simulink model "Robot_DH_FK"  (R2023b)
settings: Solver=VariableStepAuto  StartTime=0.0  StopTime=10.0  RelTol=1e-3
values from neighbouring files (symbols this model uses):
  a1 = 40    [FK.m]    (also in IK_Analytical.m = 0.04; IK_MDH.m = 0.04; IK_Position.m = 0.04; IK_Solver.m = 0.04)
  a2 = 275    [FK.m]    (also in IK_Analytical.m = 0.275; IK_MDH.m = 0.275; IK_Position.m = 0.275; IK_Solver.m = 0.275)
  a3 = 25    [FK.m]    (also in IK_Analytical.m = 0.025; IK_MDH.m = 0.025; IK_Position.m = 0.025; IK_Solver.m = 0.025)
  d1 = 342    [FK.m]    (also in IK_Analytical.m = 0.342; IK_MDH.m = 0.342; IK_Position.m = 0.342; IK_Solver.m = 0.342)
  d4 = 280    [FK.m]    (also in IK_Analytical.m = 0.28; IK_MDH.m = 0.28; IK_Position.m = 0.28; IK_Solver.m = 0.28)
  fc1 = 0    [set_mode_parameter.m]
  fc2 = 0    [set_mode_parameter.m]
  fc3 = 0    [set_mode_parameter.m]
  fc4 = 0    [set_mode_parameter.m]
  fc5 = 0    [set_mode_parameter.m]
  fc6 = 0    [set_mode_parameter.m]
  fv1 = 0    [set_mode_parameter.m]
  fv2 = 0    [set_mode_parameter.m]
  fv3 = 0    [set_mode_parameter.m]
  fv4 = 0    [set_mode_parameter.m]
  fv5 = 0    [set_mode_parameter.m]
  fv6 = 0    [set_mode_parameter.m]
  Ia1 = 0    [set_mode_parameter.m]
  Ia2 = 0    [set_mode_parameter.m]
  Ia3 = 0    [set_mode_parameter.m]
  Ia4 = 0    [set_mode_parameter.m]
  Ia5 = 0    [set_mode_parameter.m]
  Ia6 = 0    [set_mode_parameter.m]
  Ic111 = 0    [set_mode_parameter.m]
  Ic112 = 0    [set_mode_parameter.m]
  Ic113 = 0    [set_mode_parameter.m]
  Ic122 = 0    [set_mode_parameter.m]
  Ic123 = 0    [set_mode_parameter.m]
  Ic133 = 1.3676    [set_mode_parameter.m]
  Ic211 = 8.8194    [set_mode_parameter.m]
  Ic212 = 0    [set_mode_parameter.m]
  Ic213 = 0    [set_mode_parameter.m]
  Ic222 = 6.0549    [set_mode_parameter.m]
  Ic223 = 0    [set_mode_parameter.m]
  Ic233 = 0.9569    [set_mode_parameter.m]
  Ic311 = 0.0332    [set_mode_parameter.m]
  Ic312 = 0    [set_mode_parameter.m]
  Ic313 = 0    [set_mode_parameter.m]
  Ic322 = 1.8442    [set_mode_parameter.m]
  Ic323 = 0    [set_mode_parameter.m]
  Ic333 = 1.0560    (= 1.056)    [set_mode_parameter.m]
  Ic411 = 0.1448    [set_mode_parameter.m]
  Ic412 = 0    [set_mode_parameter.m]
  Ic413 = 0    [set_mode_parameter.m]
  Ic422 = 0.0015    [set_mode_parameter.m]
  Ic423 = 0    [set_mode_parameter.m]
  Ic433 = 0.0822    [set_mode_parameter.m]
  Ic511 = 0    [set_mode_parameter.m]
  Ic512 = 0    [set_mode_parameter.m]
  Ic513 = 0    [set_mode_parameter.m]
  Ic522 = 0.0121    [set_mode_parameter.m]
  Ic523 = 0    [set_mode_parameter.m]
  Ic533 = 0.0299    [set_mode_parameter.m]
  Ic611 = 0.0134    [set_mode_parameter.m]
  Ic612 = 0    [set_mode_parameter.m]
  Ic613 = 0    [set_mode_parameter.m]
  Ic622 = 0    [set_mode_parameter.m]
  Ic623 = 0    [set_mode_parameter.m]
  Ic633 = 0.0051    [set_mode_parameter.m]
  m = (c1*px + s1*py) - dt*(c1*ax + s1*ay) - a1    [IK_6DOF_Robot.m]    (also in IK_MDH.m = pwx_1 - a1; IK_MDH_Robot.m = rho - a1)
  m1 = 0.167    [set_mode_parameter.m]
  m2 = 1    [set_mode_parameter.m]
  m3 = 0.5    [set_mode_parameter.m]
  m4 = 0.333    [set_mode_parameter.m]
  m5 = 0.25    [set_mode_parameter.m]
  m6 = 0.2    [set_mode_parameter.m]
  mc11 = 0    [set_mode_parameter.m]
  mc12 = 0    [set_mode_parameter.m]
  mc13 = 0.2    [set_mode_parameter.m]
  mc21 = 0.1291    [set_mode_parameter.m]
  mc22 = 0    [set_mode_parameter.m]
  mc23 = 3.3117    [set_mode_parameter.m]
  mc31 = 1.6484    [set_mode_parameter.m]
  mc32 = 0    [set_mode_parameter.m]
  mc33 = 0.8748    [set_mode_parameter.m]
  mc41 = 0.3200    (= 0.32)    [set_mode_parameter.m]
  mc42 = 0.2324    [set_mode_parameter.m]
  mc43 = 0.7083    [set_mode_parameter.m]
  mc51 = 0.4574    [set_mode_parameter.m]
  mc52 = 0    [set_mode_parameter.m]
  mc53 = 0.6427    [set_mode_parameter.m]
  mc61 = 0.3200    (= 0.32)    [set_mode_parameter.m]
  mc62 = -0.0513    [set_mode_parameter.m]
  mc63 = 0.6417    [set_mode_parameter.m]
  MDH = [ ... (first row only)    [FK_MDH.m]    (also in optimize_MDH_params.m = [x(1:6), [0; 0; 0.275; 0.025; 0; 0],         [0.342; 0.040; ; set_mode_parameter.m; test_222.m)
  N = size(waypoints, 2)    [run_trajectory.m]
  s = zc - d(1)    [inverse_kinematics_6dof.m]
  XB4 = SerialLink([L1 L2 L3 L4 L5 L6], 'name', 'XB4')    [Toolbox_Motheds_1.m]
undefined symbols (not defined in the file or in its folder): X, Y, Z
libraries: sm_lib x56, nesl_utility x31, simulink_extras x2, simulink x2, robotcorelib x1
(part 2 of 2)

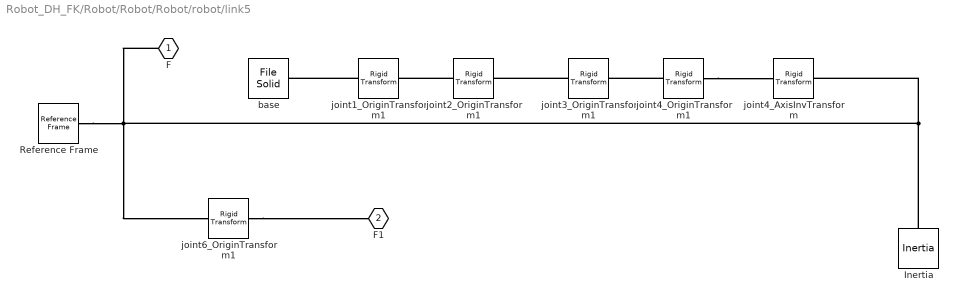
== system Robot_DH_FK/Robot/Robot/Robot/robot/link5 ==
  Inertia : sm_lib/Body Elements/Inertia  InertiaType=Custom  Mass=m5  MassUnits=kg  CenterOfMass=[mc51 mc52 mc53]  CenterOfMassUnits=m  MomentsOfInertia=[Ic511 Ic522 Ic533]  MomentsOfInertiaUnits=kg*m^2  ProductsOfInertia=[Ic523 Ic513 Ic512]  ProductsOfInertiaUnits=kg*m^2  GraphicType=Marker  MarkerShape=Inertia  MarkerSize=20  GraphicVisPropType=SimpleVisualProperties  GraphicDiffuseColor=[0.5 0.5 0.5]  GraphicSpecularColor=[0.5 0.5 0.5 1.0]  GraphicAmbientColor=[0.15 0.15 0.15 1.0]  GraphicEmissiveColor=[0.0 0.0 0.0 1.0]  GraphicShininess=75  GraphicOpacity=1.0
  Reference Frame : sm_lib/Frames and Transforms/Reference Frame
  base : sm_lib/Body Elements/File Solid  ExtGeomFileName=/home/jiehuang/Documents/Custom-Robot/Matlab_Study/Matlab2023Project/IntroductionBook/程序/XB4模型/XB4-5.STL  UnitType=Custom  ExtGeomFileUnits=mm  StepReaderType=HEX  ExportConvexHullGeometry=off  InertiaType=Custom  Mass=0  MassUnits=kg  CenterOfMass=[0 0 0]  CenterOfMassUnits=m  MomentsOfInertia=[0 0 0]  MomentsOfInertiaUnits=kg*m^2  ProductsOfInertia=[0 0 0]  ProductsOfInertiaUnits=kg*m^2  BasedOnType=Density  Density=1000  DensityUnits=kg/(m^3)  DoExposeReferenceFrame=on  SerializedFrames=<Frames/>  GraphicType=FromGeometry  MarkerShape=Sphere  MarkerSize=10  GraphicVisPropType=SimpleVisualProperties  GraphicDiffuseColor=[0.5 0.5 0.5]  GraphicSpecularColor=[0.5 0.5 0.5 1.0]  GraphicAmbientColor=[0.15 0.15 0.15 1.0]  GraphicEmissiveColor=[0.0 0.0 0.0 1.0]  GraphicShininess=75  GraphicOpacity=1.0
  joint1_OriginTransform1 : sm_lib/Frames and Transforms/Rigid Transform  TranslationMethod=Cartesian  TranslationStandardOffset=0  TranslationStandardOffsetUnits=m  TranslationStandardAxis=+Z  TranslationCartesianOffset=[0 0 d1]  TranslationCartesianOffsetUnits=m  TranslationROffset=0  TranslationROffsetUnits=m  TranslationZOffset=0  TranslationZOffsetUnits=m  TranslationThetaOffset=0  TranslationThetaOffsetUnits=deg  RotationMethod=RotationSequence  RotationAngleUnits=deg  RotationStandardAxis=+Z  RotationAngle=0.0  RotationArbitraryAxis=[0 0 1]  FollAlignAxisA=+X  BaseAlignAxisA=+Y  FollAlignAxisB=+Y  BaseAlignAxisB=+Z  RotationSequenceAxes=BaseAxes  RotationSequence=XYZ  RotationSequenceAngles=[0 0 0]  RotationSequenceAnglesUnits=rad  RotationMatrix=[1 0 0; 0 1 0; 0 0 1]  Quaternion=[1 0 0 0]
  joint2_OriginTransform1 : sm_lib/Frames and Transforms/Rigid Transform  TranslationMethod=Cartesian  TranslationStandardOffset=0  TranslationStandardOffsetUnits=m  TranslationStandardAxis=+Z  TranslationCartesianOffset=[a1 0 0]  TranslationCartesianOffsetUnits=m  TranslationROffset=0  TranslationROffsetUnits=m  TranslationZOffset=0  TranslationZOffsetUnits=m  TranslationThetaOffset=0  TranslationThetaOffsetUnits=deg  RotationMethod=RotationSequence  RotationAngleUnits=deg  RotationStandardAxis=+Z  RotationAngle=0.0  RotationArbitraryAxis=[0 0 1]  FollAlignAxisA=+X  BaseAlignAxisA=+Y  FollAlignAxisB=+Y  BaseAlignAxisB=+Z  RotationSequenceAxes=FollowerAxes  RotationSequence=XYZ  RotationSequenceAngles=[-pi/2 0 -pi/2]  RotationSequenceAnglesUnits=rad  RotationMatrix=[1 0 0; 0 1 0; 0 0 1]  Quaternion=[1 0 0 0]
  joint3_OriginTransform1 : sm_lib/Frames and Transforms/Rigid Transform  TranslationMethod=Cartesian  TranslationStandardOffset=0  TranslationStandardOffsetUnits=m  TranslationStandardAxis=+Z  TranslationCartesianOffset=[a2 0 0]  TranslationCartesianOffsetUnits=m  TranslationROffset=0  TranslationROffsetUnits=m  TranslationZOffset=0  TranslationZOffsetUnits=m  TranslationThetaOffset=0  TranslationThetaOffsetUnits=deg  RotationMethod=RotationSequence  RotationAngleUnits=deg  RotationStandardAxis=+Z  RotationAngle=0.0  RotationArbitraryAxis=[0 0 1]  FollAlignAxisA=+X  BaseAlignAxisA=+Y  FollAlignAxisB=+Y  BaseAlignAxisB=+Z  RotationSequenceAxes=FollowerAxes  RotationSequence=XYZ  RotationSequenceAngles=[0 0 0]  RotationSequenceAnglesUnits=rad  RotationMatrix=[1 0 0; 0 1 0; 0 0 1]  Quaternion=[1 0 0 0]
  joint4_AxisInvTransform : sm_lib/Frames and Transforms/Rigid Transform  TranslationMethod=Cartesian  TranslationStandardOffset=0  TranslationStandardOffsetUnits=m  TranslationStandardAxis=+Z  TranslationCartesianOffset=[0 0 0]  TranslationCartesianOffsetUnits=m  TranslationROffset=0  TranslationROffsetUnits=m  TranslationZOffset=0  TranslationZOffsetUnits=m  TranslationThetaOffset=0  TranslationThetaOffsetUnits=deg  RotationMethod=RotationSequence  RotationAngleUnits=rad  RotationStandardAxis=+Z  RotationAngle=1.570796  RotationArbitraryAxis=[0 1 0]  FollAlignAxisA=+X  BaseAlignAxisA=+Y  FollAlignAxisB=+Y  BaseAlignAxisB=+Z  RotationSequenceAxes=FollowerAxes  RotationSequence=XYZ  RotationSequenceAngles=[pi/2 0 0]  RotationSequenceAnglesUnits=rad  RotationMatrix=[1 0 0; 0 1 0; 0 0 1]  Quaternion=[1 0 0 0]
  joint4_OriginTransform1 : sm_lib/Frames and Transforms/Rigid Transform  TranslationMethod=Cartesian  TranslationStandardOffset=0  TranslationStandardOffsetUnits=m  TranslationStandardAxis=+Z  TranslationCartesianOffset=[a3 d4 0]  TranslationCartesianOffsetUnits=m  TranslationROffset=0  TranslationROffsetUnits=m  TranslationZOffset=0  TranslationZOffsetUnits=m  TranslationThetaOffset=0  TranslationThetaOffsetUnits=deg  RotationMethod=RotationSequence  RotationAngleUnits=deg  RotationStandardAxis=+Z  RotationAngle=0.0  RotationArbitraryAxis=[0 0 1]  FollAlignAxisA=+X  BaseAlignAxisA=+Y  FollAlignAxisB=+Y  BaseAlignAxisB=+Z  RotationSequenceAxes=FollowerAxes  RotationSequence=XYZ  RotationSequenceAngles=[-pi/2 0 0]  RotationSequenceAnglesUnits=rad  RotationMatrix=[1 0 0; 0 1 0; 0 0 1]  Quaternion=[1 0 0 0]
  joint6_OriginTransform1 : sm_lib/Frames and Transforms/Rigid Transform  TranslationMethod=Cartesian  TranslationStandardOffset=0  TranslationStandardOffsetUnits=m  TranslationStandardAxis=+Z  TranslationCartesianOffset=[0 0 0]  TranslationCartesianOffsetUnits=m  TranslationROffset=0  TranslationROffsetUnits=m  TranslationZOffset=0  TranslationZOffsetUnits=m  TranslationThetaOffset=0  TranslationThetaOffsetUnits=deg  RotationMethod=RotationSequence  RotationAngleUnits=deg  RotationStandardAxis=+Z  RotationAngle=0.0  RotationArbitraryAxis=[0 0 1]  FollAlignAxisA=+X  BaseAlignAxisA=+Y  FollAlignAxisB=+Y  BaseAlignAxisB=+Z  RotationSequenceAxes=FollowerAxes  RotationSequence=XYZ  RotationSequenceAngles=[-pi/2 0 0]  RotationSequenceAnglesUnits=rad  RotationMatrix=[1 0 0; 0 1 0; 0 0 1]  Quaternion=[1 0 0 0]
  F : PMIOPort  Side=Left
  F1 : PMIOPort  Port=2  Side=Right
  connections:
  Reference Frame/RConn1 -- Inertia/RConn1 -- joint4_AxisInvTransform/RConn1 -- F/RConn1 -- joint6_OriginTransform1/LConn1
  joint6_OriginTransform1/RConn1 -- F1/RConn1
  joint1_OriginTransform1/LConn1 -- base/RConn1
  joint3_OriginTransform1/LConn1 -- joint2_OriginTransform1/RConn1
  joint4_OriginTransform1/LConn1 -- joint3_OriginTransform1/RConn1
  joint2_OriginTransform1/LConn1 -- joint1_OriginTransform1/RConn1
  joint4_OriginTransform1/RConn1 -- joint4_AxisInvTransform/LConn1

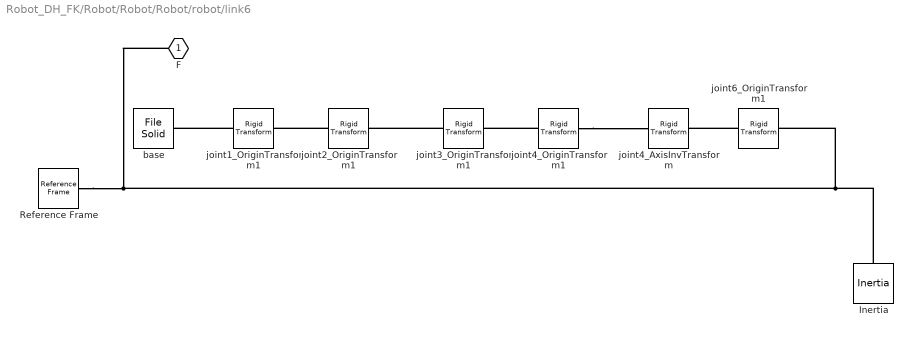
== system Robot_DH_FK/Robot/Robot/Robot/robot/link6 ==
  Inertia : sm_lib/Body Elements/Inertia  InertiaType=Custom  Mass=m6  MassUnits=kg  CenterOfMass=[mc61 mc62 mc63]  CenterOfMassUnits=m  MomentsOfInertia=[Ic611 Ic622 Ic633 ]  MomentsOfInertiaUnits=kg*m^2  ProductsOfInertia=[Ic623 Ic613 Ic612]  ProductsOfInertiaUnits=kg*m^2  GraphicType=Marker  MarkerShape=Inertia  MarkerSize=20  GraphicVisPropType=SimpleVisualProperties  GraphicDiffuseColor=[0.5 0.5 0.5]  GraphicSpecularColor=[0.5 0.5 0.5 1.0]  GraphicAmbientColor=[0.15 0.15 0.15 1.0]  GraphicEmissiveColor=[0.0 0.0 0.0 1.0]  GraphicShininess=75  GraphicOpacity=1.0
  Reference Frame : sm_lib/Frames and Transforms/Reference Frame
  base : sm_lib/Body Elements/File Solid  ExtGeomFileName=/home/jiehuang/Documents/Custom-Robot/Matlab_Study/Matlab2023Project/IntroductionBook/程序/XB4模型/XB4-6.STL  UnitType=Custom  ExtGeomFileUnits=mm  StepReaderType=HEX  ExportConvexHullGeometry=off  InertiaType=Custom  Mass=0  MassUnits=kg  CenterOfMass=[0 0 0]  CenterOfMassUnits=m  MomentsOfInertia=[0 0 0]  MomentsOfInertiaUnits=kg*m^2  ProductsOfInertia=[0 0 0]  ProductsOfInertiaUnits=kg*m^2  BasedOnType=Density  Density=1000  DensityUnits=kg/(m^3)  DoExposeReferenceFrame=on  SerializedFrames=<Frames/>  GraphicType=FromGeometry  MarkerShape=Sphere  MarkerSize=10  GraphicVisPropType=SimpleVisualProperties  GraphicDiffuseColor=[0.5 0.5 0.5]  GraphicSpecularColor=[0.5 0.5 0.5 1.0]  GraphicAmbientColor=[0.15 0.15 0.15 1.0]  GraphicEmissiveColor=[0.0 0.0 0.0 1.0]  GraphicShininess=75  GraphicOpacity=1.0
  joint1_OriginTransform1 : sm_lib/Frames and Transforms/Rigid Transform  TranslationMethod=Cartesian  TranslationStandardOffset=0  TranslationStandardOffsetUnits=m  TranslationStandardAxis=+Z  TranslationCartesianOffset=[0 0 d1]  TranslationCartesianOffsetUnits=m  TranslationROffset=0  TranslationROffsetUnits=m  TranslationZOffset=0  TranslationZOffsetUnits=m  TranslationThetaOffset=0  TranslationThetaOffsetUnits=deg  RotationMethod=RotationSequence  RotationAngleUnits=deg  RotationStandardAxis=+Z  RotationAngle=0.0  RotationArbitraryAxis=[0 0 1]  FollAlignAxisA=+X  BaseAlignAxisA=+Y  FollAlignAxisB=+Y  BaseAlignAxisB=+Z  RotationSequenceAxes=BaseAxes  RotationSequence=XYZ  RotationSequenceAngles=[0 0 0]  RotationSequenceAnglesUnits=rad  RotationMatrix=[1 0 0; 0 1 0; 0 0 1]  Quaternion=[1 0 0 0]
  joint2_OriginTransform1 : sm_lib/Frames and Transforms/Rigid Transform  TranslationMethod=Cartesian  TranslationStandardOffset=0  TranslationStandardOffsetUnits=m  TranslationStandardAxis=+Z  TranslationCartesianOffset=[a1 0 0]  TranslationCartesianOffsetUnits=m  TranslationROffset=0  TranslationROffsetUnits=m  TranslationZOffset=0  TranslationZOffsetUnits=m  TranslationThetaOffset=0  TranslationThetaOffsetUnits=deg  RotationMethod=RotationSequence  RotationAngleUnits=deg  RotationStandardAxis=+Z  RotationAngle=0.0  RotationArbitraryAxis=[0 0 1]  FollAlignAxisA=+X  BaseAlignAxisA=+Y  FollAlignAxisB=+Y  BaseAlignAxisB=+Z  RotationSequenceAxes=FollowerAxes  RotationSequence=XYZ  RotationSequenceAngles=[-pi/2 0 -pi/2]  RotationSequenceAnglesUnits=rad  RotationMatrix=[1 0 0; 0 1 0; 0 0 1]  Quaternion=[1 0 0 0]
  joint3_OriginTransform1 : sm_lib/Frames and Transforms/Rigid Transform  TranslationMethod=Cartesian  TranslationStandardOffset=0  TranslationStandardOffsetUnits=m  TranslationStandardAxis=+Z  TranslationCartesianOffset=[a2 0 0]  TranslationCartesianOffsetUnits=m  TranslationROffset=0  TranslationROffsetUnits=m  TranslationZOffset=0  TranslationZOffsetUnits=m  TranslationThetaOffset=0  TranslationThetaOffsetUnits=deg  RotationMethod=RotationSequence  RotationAngleUnits=deg  RotationStandardAxis=+Z  RotationAngle=0.0  RotationArbitraryAxis=[0 0 1]  FollAlignAxisA=+X  BaseAlignAxisA=+Y  FollAlignAxisB=+Y  BaseAlignAxisB=+Z  RotationSequenceAxes=FollowerAxes  RotationSequence=XYZ  RotationSequenceAngles=[0 0 0]  RotationSequenceAnglesUnits=rad  RotationMatrix=[1 0 0; 0 1 0; 0 0 1]  Quaternion=[1 0 0 0]
  joint4_AxisInvTransform : sm_lib/Frames and Transforms/Rigid Transform  TranslationMethod=Cartesian  TranslationStandardOffset=0  TranslationStandardOffsetUnits=m  TranslationStandardAxis=+Z  TranslationCartesianOffset=[0 0 0]  TranslationCartesianOffsetUnits=m  TranslationROffset=0  TranslationROffsetUnits=m  TranslationZOffset=0  TranslationZOffsetUnits=m  TranslationThetaOffset=0  TranslationThetaOffsetUnits=deg  RotationMethod=RotationSequence  RotationAngleUnits=rad  RotationStandardAxis=+Z  RotationAngle=1.570796  RotationArbitraryAxis=[0 1 0]  FollAlignAxisA=+X  BaseAlignAxisA=+Y  FollAlignAxisB=+Y  BaseAlignAxisB=+Z  RotationSequenceAxes=FollowerAxes  RotationSequence=XYZ  RotationSequenceAngles=[pi/2 0 0]  RotationSequenceAnglesUnits=rad  RotationMatrix=[1 0 0; 0 1 0; 0 0 1]  Quaternion=[1 0 0 0]
  joint4_OriginTransform1 : sm_lib/Frames and Transforms/Rigid Transform  TranslationMethod=Cartesian  TranslationStandardOffset=0  TranslationStandardOffsetUnits=m  TranslationStandardAxis=+Z  TranslationCartesianOffset=[a3 d4 0]  TranslationCartesianOffsetUnits=m  TranslationROffset=0  TranslationROffsetUnits=m  TranslationZOffset=0  TranslationZOffsetUnits=m  TranslationThetaOffset=0  TranslationThetaOffsetUnits=deg  RotationMethod=RotationSequence  RotationAngleUnits=deg  RotationStandardAxis=+Z  RotationAngle=0.0  RotationArbitraryAxis=[0 0 1]  FollAlignAxisA=+X  BaseAlignAxisA=+Y  FollAlignAxisB=+Y  BaseAlignAxisB=+Z  RotationSequenceAxes=FollowerAxes  RotationSequence=XYZ  RotationSequenceAngles=[-pi/2 0 0]  RotationSequenceAnglesUnits=rad  RotationMatrix=[1 0 0; 0 1 0; 0 0 1]  Quaternion=[1 0 0 0]
  joint6_OriginTransform1 : sm_lib/Frames and Transforms/Rigid Transform  TranslationMethod=Cartesian  TranslationStandardOffset=0  TranslationStandardOffsetUnits=m  TranslationStandardAxis=+Z  TranslationCartesianOffset=[0 0 0]  TranslationCartesianOffsetUnits=m  TranslationROffset=0  TranslationROffsetUnits=m  TranslationZOffset=0  TranslationZOffsetUnits=m  TranslationThetaOffset=0  TranslationThetaOffsetUnits=deg  RotationMethod=RotationSequence  RotationAngleUnits=deg  RotationStandardAxis=+Z  RotationAngle=0.0  RotationArbitraryAxis=[0 0 1]  FollAlignAxisA=+X  BaseAlignAxisA=+Y  FollAlignAxisB=+Y  BaseAlignAxisB=+Z  RotationSequenceAxes=FollowerAxes  RotationSequence=XYZ  RotationSequenceAngles=[-pi/2 0 0]  RotationSequenceAnglesUnits=rad  RotationMatrix=[1 0 0; 0 1 0; 0 0 1]  Quaternion=[1 0 0 0]
  F : PMIOPort  Side=Left
  connections:
  Reference Frame/RConn1 -- joint6_OriginTransform1/RConn1 -- Inertia/RConn1 -- F/RConn1
  joint6_OriginTransform1/LConn1 -- joint4_AxisInvTransform/RConn1
  joint1_OriginTransform1/LConn1 -- base/RConn1
  joint3_OriginTransform1/LConn1 -- joint2_OriginTransform1/RConn1
  joint4_OriginTransform1/RConn1 -- joint4_AxisInvTransform/LConn1
  joint4_OriginTransform1/LConn1 -- joint3_OriginTransform1/RConn1
  joint2_OriginTransform1/LConn1 -- joint1_OriginTransform1/RConn1

== matlab function Robot_DH_FK/MATLAB Function ==
  data: Radian input; KPS44 output
function KPS44 = FK_DH(Radian)
% FK using Standard DH parameters (替代原MDH)
% 输入:  Radian[1x6] 六个关节角 (rad)
% 输出:  KPS44[4x4] 末端在基坐标系下的齐次变换矩阵 (m)
%
% 零位姿: [0 0 1 0.393; 0 -1 0 0; 1 0 0 0.642; 0 0 0 1]
% 标准DH参数（对应XB4）:
% 关节i: theta_i(输入+偏移) | d_i    | a_i     | alpha_i
%  1    : Radian(1)        | 0.342  | 0.040   | -pi/2
%  2    : Radian(2)-pi/2   | 0      | 0.275   | 0
%  3    : Radian(3)        | 0      | 0.025   | -pi/2
%  4    : Radian(4)        | 0.280  | 0       | pi/2
%  5    : Radian(5)        | 0      | 0       | -pi/2
%  6    : Radian(6)        | 0.073  | 0       | 0

theta = Radian(:);  % 转为列向量

%% 标准DH参数表 (单位: m, rad)
% 每行: [alpha_i, a_i, d_i, theta_offset]
DH = [
    -pi/2,    0.040,    0.342,    0;      % 关节1
     0,       0.275,    0,        -pi/2;   % 关节2 (theta偏移-pi/2)
    -pi/2,    0.025,    0,        0;      % 关节3
     pi/2,    0,        0.280,    0;      % 关节4
    -pi/2,    0,        0,        0;      % 关节5
     0,       0,        0.073,    0;      % 关节6
];

%% 正运动学计算（标准DH）
T = eye(4);  % 初始化为单位矩阵（基坐标系->0号坐标系）

for i = 1:6
    alpha = DH(i,1);  % alpha_i: 绕X_i旋转角度
    a     = DH(i,2);  % a_i: 沿X_i平移距离
    d     = DH(i,3);  % d_i: 沿Z_{i-1}平移距离
    offset= DH(i,4);  % theta_i的偏移量
    
    theta_i = theta(i) + offset;  % 最终关节角（输入+偏移）
    
    % 标准DH变换矩阵公式
    % T_{i-1,i} = Rot(Z_{i-1}, θ_i) * Trans(Z_{i-1}, d_i) * Trans(X_i, a_i) * Rot(X_i, α_i)
    ct = cos(theta_i);
    st = sin(theta_i);
    ca = cos(alpha);
    sa = sin(alpha);
    
    T_i = [ct,   -st*ca,    st*sa,   a*ct;
           st,    ct*ca,   -ct*sa,   a*st;
           0,      sa,       ca,      d;
           0,      0,        0,       1];
    
    T = T * T_i;  % 累积变换（基坐标系->i号坐标系）
end

KPS44 = T;
end

== matlab function Robot_DH_FK/Robot/Robot/Robot/robot/Jm ==
  data: u input; y output; Jm input
function y = fcn(u,Jm)
%#codegen

% Jm=[200; 250; 150; 100; 50; 20];%关节惯性
y = Jm.*u;
end

== matlab function Robot_DH_FK/Robot/Robot/Robot/robot/friction ==
  data: u input; y output; fv input; fc input
function y = fcn(u,fv,fc)
%#codegen


% fv1=100; fc1=80; fv2=150; fc2=100; fv3=100; fc3=50; fv4=80; fc4=80; fv5=50; fc5=30; fv6=30; fc6=10;
fv1=fv(1); fc1=fc(1); fv2=fv(2); fc2=fc(2); fv3=fv(3); fc3=fc(3); fv4=fv(4); fc4=fc(4); fv5=fv(5); fc5=fc(5); fv6=fv(6); fc6=fc(6);
y=[0;0;0;0;0;0];
y(1)=(fv1*u(1)+fc1*sign(u(1)));
y(2)=(fv2*u(2)+fc2*sign(u(2)));
y(3)=(fv3*u(3)+fc3*sign(u(3)));
y(4)=(fv4*u(4)+fc4*sign(u(4)));
y(5)=(fv5*u(5)+fc5*sign(u(5)));
y(6)=(fv6*u(6)+fc6*sign(u(6)));

end
